simulink model "qq1"  (R2020a)
settings: Solver=VariableStepAuto  StartTime=0.0  StopTime=10.0  RelTol=1e-3
undefined symbols (not defined in the file): B, K1, K2, M1, M2
settings Model: Creator=kiran  LastModifiedBy=kiran

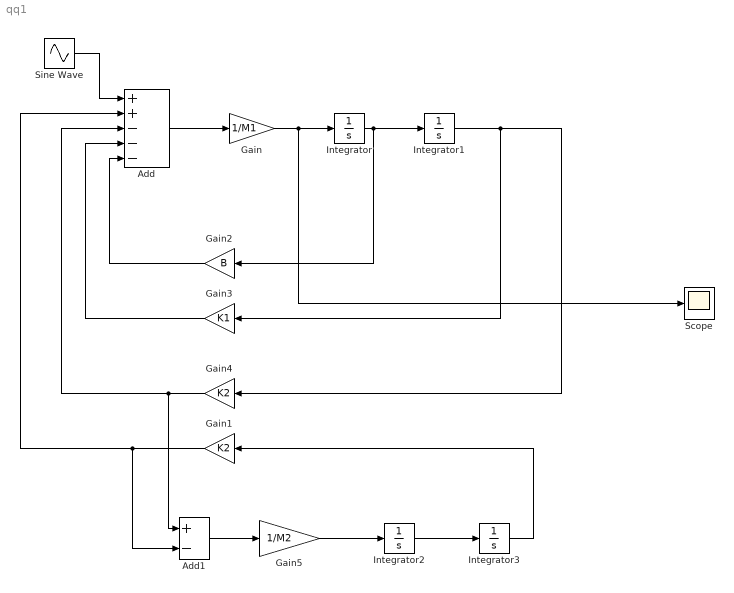
== system qq1 ==
  Add : Sum  Inputs=++---
  Add1 : Sum  Inputs=+-
  Gain : Gain  Gain=1/M1
  Gain1 : Gain  Gain=K2
  Gain2 : Gain  Gain=B
  Gain3 : Gain  Gain=K1
  Gain4 : Gain  Gain=K2
  Gain5 : Gain  Gain=1/M2
  Integrator{,1..3} (4 alike) : Integrator
  Scope : Scope
  Sine Wave : Sin  Amplitude=2  Frequency=10  SampleTime=0
  wires:
  Integrator/1 -> Gain2/1, Integrator1/1
  Gain/1 -> Scope/1, Integrator/1
  Add1/1 -> Gain5/1
  Gain3/1 -> Add/4
  Gain4/1 -> Add1/1, Add/3
  Gain2/1 -> Add/5
  Gain5/1 -> Integrator2/1
  Integrator1/1 -> Gain3/1, Gain4/1
  Integrator2/1 -> Integrator3/1
  Integrator3/1 -> Gain1/1
  Sine Wave/1 -> Add/1
  Add/1 -> Gain/1
  Gain1/1 -> Add1/2, Add/2
